simulink model "nonlinear"  (R2016b)
settings: Solver=VariableStepAuto  StartTime=0.0  StopTime=10.0  RelTol=1e-3
settings Model: Creator=tangxiaoli  LastModifiedBy=tangxiaoli

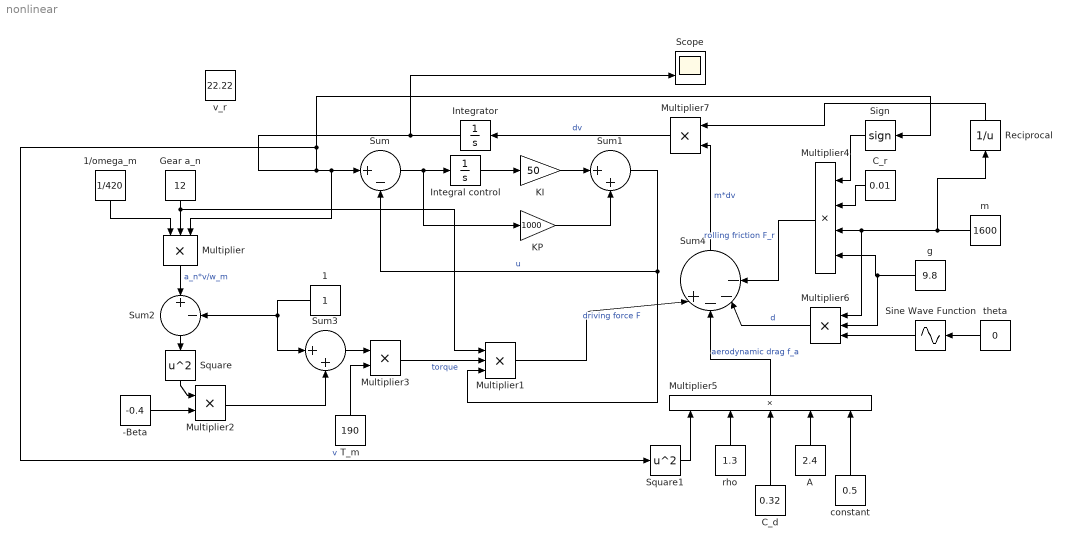
== system nonlinear ==
  -Beta : Constant  Value=-0.4
  1 : Constant
  1/omega_m : Constant  Value=1/420
  A : Constant  Value=2.4
  C_d : Constant  Value=0.32
  C_r : Constant  Value=0.01
  Gear a_n : Constant  Value=12
  Integral control : Integrator
  Integrator : Integrator
  KI : Gain  Gain=50
  KP : Gain  Gain=1000
  Multiplier : Product  Inputs=***
  Multiplier1 : Product  Inputs=***
  Multiplier2 : Product  Inputs=**
  Multiplier3 : Product  Inputs=**
  Multiplier4 : Product  Inputs=****
  Multiplier5 : Product  Inputs=*****
  Multiplier6 : Product  Inputs=***
  Multiplier7 : Product  Inputs=**
  "Reciprocal " : Math  Operator=reciprocal  SaturateOnIntegerOverflow=on
  Scope : Scope  NumInputPorts=2
  Sign : Signum
  Sine Wave Function : Sin  TimeSource=Use external signal  SampleTime=0
  Square : Math  Operator=square  SaturateOnIntegerOverflow=on
  Square1 : Math  Operator=square  SaturateOnIntegerOverflow=on
  Sum : Sum  Inputs=|+-
  Sum1 : Sum  Inputs=|++
  Sum2 : Sum  Inputs=|+-
  Sum3 : Sum  Inputs=|++
  Sum4 : Sum  Inputs=|+---
  T_m : Constant  Value=190
  constant : Constant  Value=0.5
  g : Constant  Value=9.8
  m : Constant  Value=1600
  rho : Constant  Value=1.3
  theta : Constant  Value=0
  v_r : Constant  Value=22.22
  wires:
  Integrator/1 -> Scope/2, Square1/1, Sign/1, Multiplier/3, Sum/1  "v"
  Sum/1 -> KP/1, Integral control/1
  KP/1 -> Sum1/2
  Integral control/1 -> KI/1
  KI/1 -> Sum1/1
  Sum1/1 -> Sum/2, Multiplier1/3  "u"
  Gear a_n/1 -> Multiplier/2, Multiplier1/1
  1/omega_m/1 -> Multiplier/1
  Multiplier/1 -> Sum2/1  "a_n*v/w_m"
  1/1 -> Sum3/1, Sum2/2
  Sum2/1 -> Square/1
  Square/1 -> Multiplier2/1
  -Beta/1 -> Multiplier2/2
  Multiplier2/1 -> Sum3/2
  Sum3/1 -> Multiplier3/1
  T_m/1 -> Multiplier3/2
  Multiplier3/1 -> Multiplier1/2  "torque"
  Multiplier1/1 -> Sum4/1  "driving force F"
  Sign/1 -> Multiplier4/1
  C_r/1 -> Multiplier4/2
  m/1 -> "Reciprocal "/1, Multiplier6/1, Multiplier4/3
  g/1 -> Multiplier6/2, Multiplier4/4
  Multiplier4/1 -> Sum4/4  "rolling friction F_r"
  Square1/1 -> Multiplier5/1
  rho/1 -> Multiplier5/2
  C_d/1 -> Multiplier5/3
  A/1 -> Multiplier5/4
  constant/1 -> Multiplier5/5
  theta/1 -> Sine Wave Function/1
  Sine Wave Function/1 -> Multiplier6/3
  Multiplier6/1 -> Sum4/3  "d"
  Multiplier5/1 -> Sum4/2  "aerodynamic drag f_a"
  Sum4/1 -> Multiplier7/2  "m*dv"
  "Reciprocal "/1 -> Multiplier7/1
  Multiplier7/1 -> Integrator/1  "dv"
